simulink model "rectifier_6T_RLE_refactor"  (R2025a)
settings: Solver=VariableStepAuto  StartTime=0.0  StopTime=0.3  RelTol=1e-3
undefined symbols (not defined in the file): alpha_deg, enable, Eo, f_grid, Lk, Lo, Ls, offset_deg, pulse_width_deg, Ro, Rs, U_LL
libraries: spsThyristorLib x6, spsThreePhaseSeriesRLCBranchLib x2, spsDCVoltageSourceLib x1, spsSeriesRLCBranchLib x1, spsThreePhaseSourceLib x1, spsCurrentMeasurementLib x1, sps_lib x1, spsVoltageMeasurementLib x1
settings Model: Creator=speed  LastModifiedBy=speed

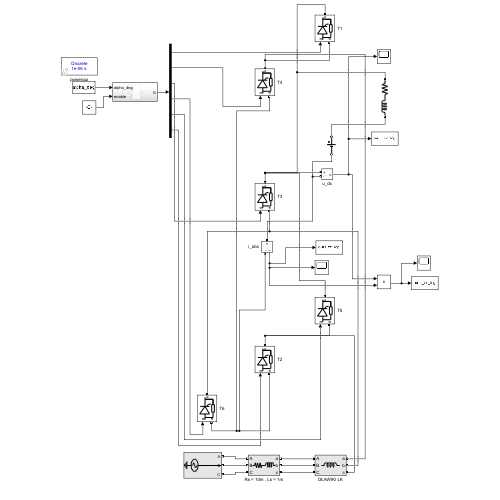
[thumbnail: Simulink's stored preview of the top-level diagram]
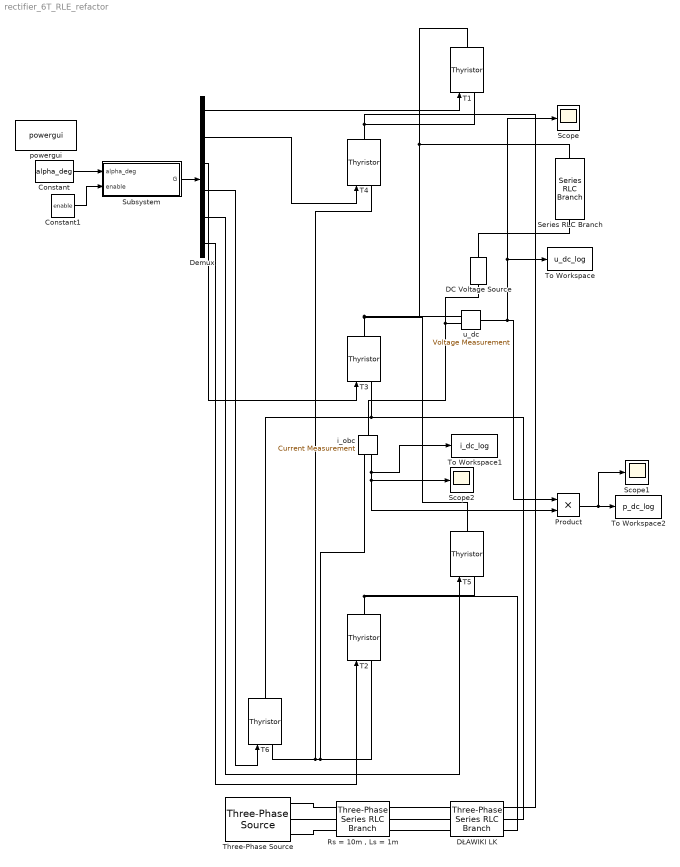
== system rectifier_6T_RLE_refactor ==
  Constant : Constant  Value=alpha_deg
  Constant1 : Constant  Value=enable
  DC Voltage Source : spsDCVoltageSourceLib/DC Voltage Source  Amplitude=Eo  Measurements=None
  Demux : Demux  Outputs=6
  DŁAWIKI LK : spsThreePhaseSeriesRLCBranchLib/Three-Phase Series RLC Branch  LConnTagsString=A|B|C  RConnTagsString=A|B|C  BranchType=L  Resistance=10e-3  Inductance=Lk  Capacitance=1e-6  Measurements=None
  Product : Product
  "Rs = 10m , Ls = 1m" : spsThreePhaseSeriesRLCBranchLib/Three-Phase Series RLC Branch  LConnTagsString=A|B|C  RConnTagsString=A|B|C  BranchType=RL  Resistance=Rs  Inductance=Ls  Capacitance=1e-6  Measurements=None
  Scope : Scope
      settings: ActiveDisplayYMinimum=-511.26816749369158  ActiveDisplayYMaximum=124.17018209541524
  Scope1 : Scope
      settings: ActiveDisplayYMinimum=-21740.759527723938  ActiveDisplayYMaximum=2443.0354714008081
  Scope2 : Scope
      settings: ActiveDisplayYMinimum=-6.8671455486357758  ActiveDisplayYMaximum=61.288741838981075  DataLoggingVariableName=ScopeData2
  Series RLC Branch : spsSeriesRLCBranchLib/Series RLC Branch  LConnTagsString=__new0  RConnTagsString=__new0  BranchType=RL  Resistance=Ro  Inductance=Lo  SetiL0=off  InitialCurrent=0  Capacitance=1e-6  Setx0=off  InitialVoltage=0  Measurements=None
  Subsystem : Subsystem
  T{1..6} (6 alike) : spsThyristorLib/Thyristor  Ron=0.001  Lon=0  Vf=0.8  IC=0  Rs=500  Cs=250e-9  Measurements=off
  Three-Phase Source : spsThreePhaseSourceLib/Three-Phase Source  InternalConnection=Yg  VoltagePhases=off  Voltage=U_LL  PhaseAngle=0  Voltage_phases=[25e3 25e3 25e3]/sqrt(3)  PhaseAngles_phases=[0 -120 +120]  Frequency=f_grid  NonIdealSource=off  SpecifyImpedance=off  Resistance=0.8929  Inductance=16.58e-3  ShortCircuitLevel=100e6  BaseVoltage=25e3  XRratio=7  BusType=swing  Pref=10e3  Qref=0  Prefabc=[10e3, 10e3, 10e3]  Qrefabc=[0, 0, 0]  Qmin=-inf  Qmax=inf
  To Workspace : ToWorkspace  VariableName=u_dc_log  SaveFormat=Timeseries  SampleTime=-1
  To Workspace1 : ToWorkspace  VariableName=i_dc_log  SaveFormat=Timeseries  SampleTime=-1
  To Workspace2 : ToWorkspace  VariableName=p_dc_log  SaveFormat=Timeseries  SampleTime=-1
  i_obc : spsCurrentMeasurementLib/Current Measurement  PhasorSimulation=off  OutputType=Complex  PSBequivalent=0
  powergui : sps_lib/powergui  Priority=1  SimulationMode=Discrete  SampleTime=1e-6  frequency=60  Iterations=50  frequencyindice=0  Pbase=100e6  ErrMax=1e-4  UnitsV=kV  UnitsW=MW  buscounter=0  FunctionMessages=off  echomessages=off  EnableUseOfTLC=off  CurrentSourceSwitches=off  DisableSnubberDevices=off  DisableRonSwitches=off  DisableVfSwitches=off  DisplayEquations=off  AutomaticDiscreteSolvers=off  SolverType=Tustin/Backward Euler (TBE)  Interpol=off  ExternalGateDelay=off  methode=off  Ts=100  x0status=blocks  SPID=on  SwTol=0  HookPort=off  NonlinearTolerance=1e-4  nMaxIteration=100  ContinueOnMaxIteration=off  RestoreLinks=warning  ResistiveCurrentMeasurement=off  Frange=[0:2:500]  Ylog=off  Xlog=on  ShowGrid=off  save=off  variable=ZData  structure=0  ZoomFFT=off  StartTime=0.0  cycles=1  DisplayStyle=1  fundamental=60  FreqAxis=off  MaxFrequency=1000  frequencyindicesteady=1  RmsSteady=1  display=off
  u_dc : spsVoltageMeasurementLib/Voltage Measurement  PhasorSimulation=off  OutputType=Complex  PSBequivalent=0
  wires:
  Demux/2 -> T4/1
  Constant/1 -> Subsystem/1(alpha_deg)
  Demux/1 -> T1/1
  Constant1/1 -> Subsystem/2(enable)
  Subsystem/1(G) -> Demux/1
  Product/1 -> Scope1/1, To Workspace2/1
  Demux/5 -> T5/1
  Demux/4 -> T6/1
  Demux/3 -> T3/1
  Demux/6 -> T2/1
  i_obc/1 -> Scope2/1, Product/2, To Workspace1/1
  u_dc/1 -> To Workspace/1, Scope/1, Product/1
  connections:
  DC Voltage Source/RConn1 -- Series RLC Branch/RConn1
  T6/LConn1 -- T2/LConn1 -- i_obc/RConn1 -- T4/LConn1
  T3/RConn1 -- Series RLC Branch/LConn1 -- T1/RConn1 -- u_dc/LConn1 -- T5/RConn1
  T4/RConn1 -- T1/LConn1 -- DŁAWIKI LK/RConn1
  T6/RConn1 -- T3/LConn1 -- DŁAWIKI LK/RConn2
  Three-Phase Source/RConn1 -- "Rs = 10m , Ls = 1m"/LConn1
  Three-Phase Source/RConn2 -- "Rs = 10m , Ls = 1m"/LConn2
  Three-Phase Source/RConn3 -- "Rs = 10m , Ls = 1m"/LConn3
  i_obc/LConn1 -- u_dc/LConn2 -- DC Voltage Source/LConn1
  T2/RConn1 -- DŁAWIKI LK/RConn3 -- T5/LConn1
  "Rs = 10m , Ls = 1m"/RConn1 -- DŁAWIKI LK/LConn1
  "Rs = 10m , Ls = 1m"/RConn2 -- DŁAWIKI LK/LConn2
  "Rs = 10m , Ls = 1m"/RConn3 -- DŁAWIKI LK/LConn3

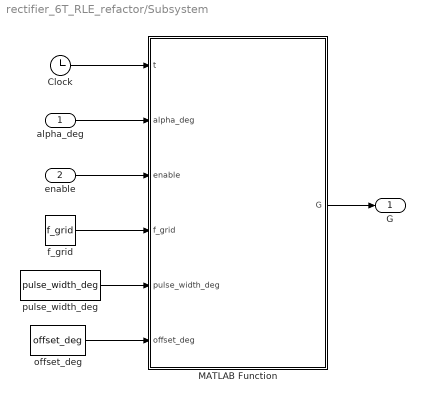
== system rectifier_6T_RLE_refactor/Subsystem ==
  alpha_deg : Inport
  enable : Inport  Port=2
  Clock : Clock
  MATLAB Function : MATLAB Function  TreatAsAtomicUnit=on
  f_grid : Constant  Value=f_grid
  offset_deg : Constant  Value=offset_deg
  pulse_width_deg : Constant  Value=pulse_width_deg
  G : Outport
  wires:
  offset_deg/1 -> MATLAB Function/6(offset_deg)
  pulse_width_deg/1 -> MATLAB Function/5(pulse_width_deg)
  alpha_deg/1 -> MATLAB Function/2(alpha_deg)
  Clock/1 -> MATLAB Function/1(t)
  f_grid/1 -> MATLAB Function/4(f_grid)
  enable/1 -> MATLAB Function/3(enable)
  MATLAB Function/1(G) -> G/1

== matlab function rectifier_6T_RLE_refactor/Subsystem/MATLAB Function ==
  data: t input; G output; alpha_deg input; enable input; f_grid input; pulse_width_deg input; offset_deg input
function G = gate_pulse_generator_6T(t, alpha_deg, enable, f_grid, pulse_width_deg, offset_deg)

% Generator bramek dla mostka tyrystorowego 6T.
%
% WERSJA DIAGNOSTYCZNA:
% zamiast krótkich impulsów generuje szerokie okna bramkowania.
%
% Ustaw na wejściu:
% pulse_width_deg = 120
%
% Klasyczna kolejność tyrystorów:
% T1 -> T2 -> T3 -> T4 -> T5 -> T6
%
% Twoje połączenie Demux:
% w1 -> g1
% w2 -> g4
% w3 -> g3
% w4 -> g6
% w5 -> g5
% w6 -> g2
%
% Dlatego wyjście:
% G = [g1; g4; g3; g6; g5; g2]

% ------------------------------------------------------------
% 1. Ograniczenie kąta sterowania
% ------------------------------------------------------------

if alpha_deg < 0
    alpha_deg = 0;
end

if alpha_deg > 170
    alpha_deg = 170;
end

% ------------------------------------------------------------
% 2. Kąt elektryczny sieci w stopniach
% ------------------------------------------------------------

theta = mod(360 * f_grid * t, 360);

% ------------------------------------------------------------
% 3. Dla diagnostyki wymuszamy szerokość okna 120 stopni
% ------------------------------------------------------------

gate_width_deg = pulse_width_deg;

if gate_width_deg <= 0
    gate_width_deg = 120;
end

% Na ten etap najlepiej używać dokładnie 120 stopni
% albo minimalnie mniej, np. 118 stopni.
% Jeśli na wejściu dasz 120, zostanie 120.

% ------------------------------------------------------------
% 4. Początki okien bramkowania w klasycznej kolejności:
%
% g1 = T1
% g2 = T2
% g3 = T3
% g4 = T4
% g5 = T5
% g6 = T6
% ------------------------------------------------------------

start_g1 = offset_deg + alpha_deg;
start_g2 = offset_deg + alpha_deg + 60;
start_g3 = offset_deg + alpha_deg + 120;
start_g4 = offset_deg + alpha_deg + 180;
start_g5 = offset_deg + alpha_deg + 240;
start_g6 = offset_deg + alpha_deg + 300;

start_g1 = mod(start_g1, 360);
start_g2 = mod(start_g2, 360);
start_g3 = mod(start_g3, 360);
start_g4 = mod(start_g4, 360);
start_g5 = mod(start_g5, 360);
start_g6 = mod(start_g6, 360);

% ------------------------------------------------------------
% 5. Generacja okien bramkowania
% ------------------------------------------------------------

g1 = gate_window(theta, start_g1, gate_width_deg);
g2 = gate_window(theta, start_g2, gate_width_deg);
g3 = gate_window(theta, start_g3, gate_width_deg);
g4 = gate_window(theta, start_g4, gate_width_deg);
g5 = gate_window(theta, start_g5, gate_width_deg);
g6 = gate_window(theta, start_g6, gate_width_deg);

% Blokada bramek
if enable <= 0.5
    g1 = 0;
    g2 = 0;
    g3 = 0;
    g4 = 0;
    g5 = 0;
    g6 = 0;
end

% ------------------------------------------------------------
% 6. Mapowanie pod Twoje połączenie Demuxa:
%
% w1 -> g1
% w2 -> g4
% w3 -> g3
% w4 -> g6
% w5 -> g5
% w6 -> g2
% ------------------------------------------------------------

G = zeros(6,1);

G(1) = g1;
G(2) = g4;
G(3) = g3;
G(4) = g6;
G(5) = g5;
G(6) = g2;

end


function y = gate_window(theta, start_angle, width_angle)

d = mod(theta - start_angle, 360);

if d >= 0 && d < width_angle
    y = 1;
else
    y = 0;
end

end
